simulink model "hdl_learn_stateflow"  (R2025b)
settings: Solver=FixedStepDiscrete  StartTime=0.0  StopTime=0.05  FixedStep=0.001  RelTol=1e-3
settings Model: DataTypeOverride=Off  Creator=kimsteph  LastModifiedBy=kimsteph
settings OptimizationCC: BlockReduction=off  ConditionallyExecuteInputs=off  DefaultParameterBehavior=Inlined  InheritOutputTypeSmallerThanSingle=on
settings DebuggingCC: ArtificialAlgebraicLoopMsg=error  SingleTaskRateTransMsg=error
settings HardwareCC: ProdBitPerPointer=32.0  ProdBitPerSizeT=32.0  ProdBitPerPtrDiffT=32.0  ProdLargestAtomicFloat=None  ProdIntDivRoundTo=Undefined  ProdEndianess=Unspecified  ProdWordSize=32.0  ProdHWDeviceType=ASIC/FPGA->ASIC/FPGA  TargetBitPerPointer=64.0  TargetBitPerSizeT=64.0  TargetBitPerPtrDiffT=64.0  TargetLongLongMode=on  TargetIntDivRoundTo=Zero  TargetEndianess=LittleEndian  TargetWordSize=64.0  TargetHWDeviceType=Custom Processor->MATLAB Host Computer  ProdEqTarget=off

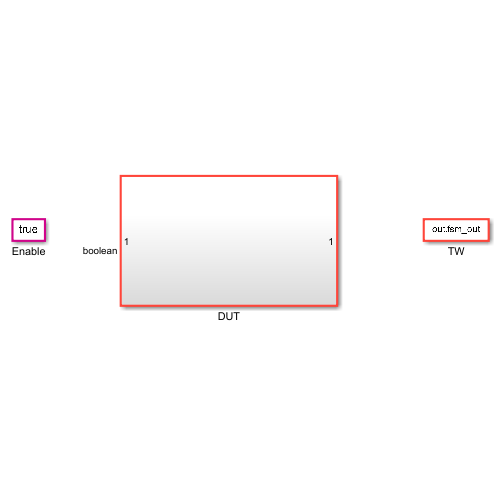
[thumbnail: Simulink's stored preview of the top-level diagram]
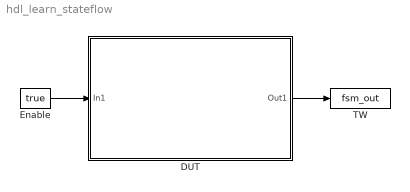
== system hdl_learn_stateflow ==
  DUT : Subsystem
  Enable : Constant  Value=true  OutDataTypeStr=boolean
  TW : ToWorkspace  VariableName=fsm_out  SaveFormat=Timeseries  SampleTime=-1
  wires:
  Enable/1 -> DUT/1(In1)
  DUT/1(Out1) -> TW/1

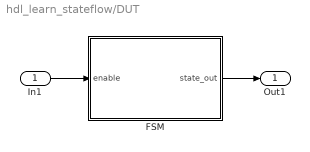
== system hdl_learn_stateflow/DUT ==
  In1 : Inport  OutDataTypeStr=boolean
  FSM : Stateflow chart  TreatAsAtomicUnit=on
  Out1 : Outport
  wires:
  In1/1 -> FSM/1(enable)
  FSM/1(state_out) -> Out1/1

== stateflow chart hdl_learn_stateflow/DUT/FSM ==
  state GREEN
    entry: state_out = uint8(0); cnt = uint16(0);
    during: cnt = cnt + uint16(1);
  state YELLOW
    entry: state_out = uint8(1); cnt = uint16(0);
    during: cnt = cnt + uint16(1);
  state RED
    entry: state_out = uint8(2); cnt = uint16(0);
    during: cnt = cnt + uint16(1);
  (default) -> GREEN
  RED -> GREEN : [cnt >= uint16(10)]
  YELLOW -> RED : [cnt >= uint16(3)]
  GREEN -> YELLOW : [cnt >= uint16(10)]
  data: enable input boolean; state_out output uint8; cnt local uint16
